simulink model "raspberrypi_edgedetect"  (R2021a)
settings: Solver=FixedStepAuto  StartTime=0.0  StopTime=inf  RelTol=1e-3  EnableMultiTasking=on
libraries: embedlinuxAVlib x1, raspberrypiAVlib x1
settings Model: Creator=The MathWorks, Inc.  LastModifiedBy=JOAKOL
settings SolverCC: AlgebraicLoopSolver=TrustRegion  PositivePriorityOrder=on
settings DataIOCC: ReturnWorkspaceOutputs=off
settings OptimizationCC: EnhancedBackFolding=on  PassReuseOutputArgsThreshold=0  MaxStackSize=64  OptimizeBlockOrder=speed  DifferentSizesBufferReuse=on  OptimizationCustomize=off
settings DebuggingCC: ParameterTunabilityLossMsg=error  SFMachineParentedDataDiag=warning  ArithmeticOperatorsInVariantConditions=warning
settings HardwareCC: ProdBitPerPointer=32  ProdBitPerSizeT=32  ProdBitPerPtrDiffT=32  ProdLargestAtomicInteger=Long  ProdLargestAtomicFloat=Double  ProdWordSize=32  ProdHWDeviceType=ARM Compatible->ARM Cortex  UseEmbeddedCoderFeatures=off  UseSimulinkCoderFeatures=off
settings SFSimCC: MATLABDynamicMemAlloc=off  CustomCodeUndefinedFunction=UseInterfaceOnly
settings RTWCC: SystemTargetFile=ert.tlc  HardwareBoard=Raspberry Pi  TLCOptions="-aInlineSetEventsForThisBaseRateFcn=TLC_FALSE -aSuppressMultiTaskScheduler=TLC_FALSE  -aRateBasedStepFcn=0"  TemplateMakefile=ert_default_tmf  GenerateReport=on  Toolchain=GNU GCC Embedded Linux  BuildConfiguration=Faster Runs  LaunchReport=on
settings CodeAppCC: ForceParamTrailComments=on  OperatorAnnotations=on
settings ERTTargetCC: ERTCustomFileBanners=off  SupportContinuousTime=on  SupportNonInlinedSFcns=on  RemoveResetFunc=off  SupportVariableSizeSignals=on  ModelStepFunctionPrototypeControlCompliant=off

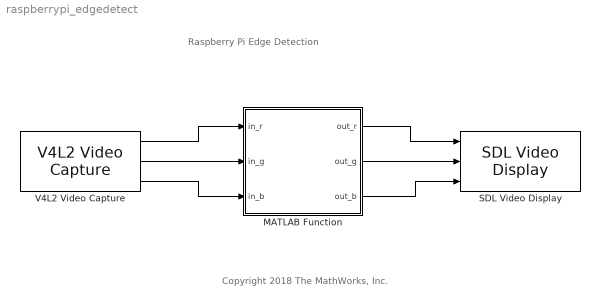
== system raspberrypi_edgedetect ==
  note: Copyright 2018 The MathWorks, Inc.
  note: Raspberry Pi Edge Detection
  MATLAB Function : MATLAB Function  TreatAsAtomicUnit=on
  SDL Video Display : embedlinuxAVlib/SDL Video Display  title=SDL Video Display  pixelFormat=RGB  pixelOrder=Planar  rowMajor=on  blockPlatform=Raspberry Pi
      settings: SourceProductBaseCode=SC_BEAGLEBONE_BLUE,NVIDIA,RASPPIIO
  V4L2 Video Capture : raspberrypiAVlib/V4L2 Video Capture  DeviceName=/dev/video0  Resolution=320x240  CustomResolution=[ 320, 240 ]  PixelFormat=RGB  SampleTime=1/10  pixelOrder=Planar  simOutput=Colorbars  imSizeSelection=320x240  imSize=[640, 480]  roi=[0, 0, 640, 480]  m_devName='/dev/video0'  blockPlatform=Raspberry Pi
      settings: SourceProductBaseCode=RASPPI
  wires:
  V4L2 Video Capture/1 -> MATLAB Function/1(in_r)
  V4L2 Video Capture/2 -> MATLAB Function/2(in_g)
  V4L2 Video Capture/3 -> MATLAB Function/3(in_b)
  MATLAB Function/1(out_r) -> SDL Video Display/1
  MATLAB Function/2(out_g) -> SDL Video Display/2
  MATLAB Function/3(out_b) -> SDL Video Display/3

== matlab function raspberrypi_edgedetect/MATLAB Function ==
  data: in_r input; out_r output; in_g input; in_b input; out_g output; out_b output
function [out_r,out_g,out_b] = edgeDetect(in_r,in_g,in_b)
%edgeDetect Edge Detection example using sobel algorithm 

%#codegen

% Copyright 2017-2018 The MathWorks, Inc.

%Define Kernel for Sobel edge detection
kern = [1 2 1; 0 0 0; -1 -2 -1];

%Frame the RGB image
img = cat(3, in_r,in_g,in_b);

%Detect Edge
h = conv2(img(:,:,2),kern,'same');
v = conv2(img(:,:,2),kern','same');
e = sqrt(h.*h + v.*v);
edgeImg = uint8((e > 100) * 240);

%output the grayscale edgeImg as a RGB image
out_r = edgeImg;
out_g = edgeImg;
out_b = edgeImg;

end
